simulink subsystem "patient_model"  (R2019b)
settings: Solver=VariableStepAuto  StartTime=0.0  StopTime=10.0  RelTol=1e-3
undefined symbols (not defined in the file): C_v_CO2_0, C_v_O2_0, Q_0
libraries: simulink x1
(part 1 of 2)
settings Model: Creator=RH  LastModifiedBy=RH

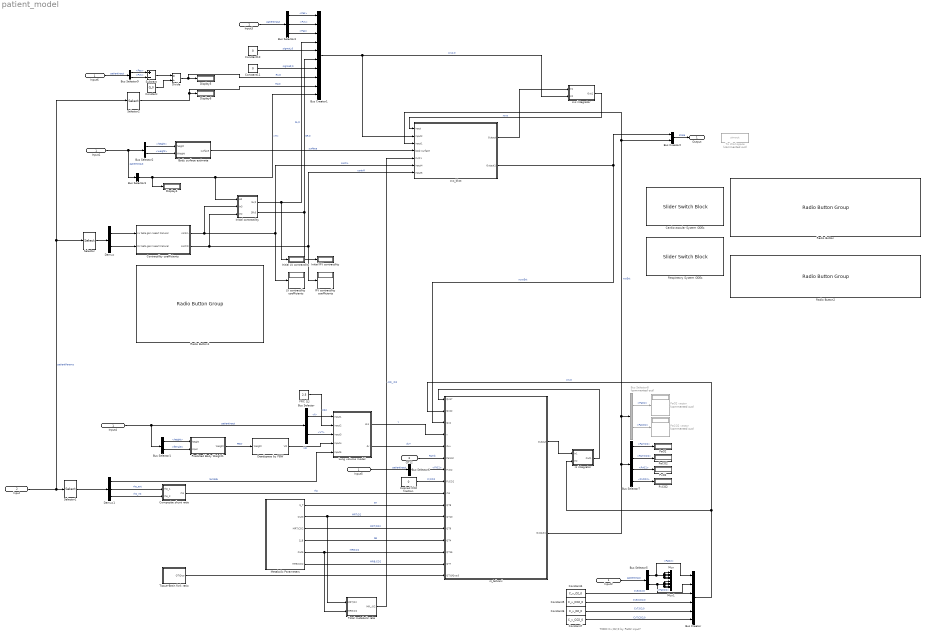
== system patient_model ==
  note: TODO Cv;O2;0 by PaO2 input?
  Input1 : Inport  OutDataTypeStr=Bus: PatientInput
  Input : Inport  Port=2  PortDimensions=6
  QT12 : Inport  Port=3  Unit=mmHg
  Body surface estimate : Subsystem  TreatAsAtomicUnit=on
  Bus Creator : BusCreator  Inputs=6  OutDataTypeStr=Bus: RespiratoryState
      settings: InheritFromInputs=off
  Bus Creator1 : BusCreator  Inputs=10  OutDataTypeStr=Bus: CardioVascularState
      settings: InheritFromInputs=off
  Bus Creator2 : BusCreator  Inputs=2  OutDataTypeStr=Bus: PatientState
      settings: InheritFromInputs=off
  Bus Selector : BusSelector  OutputSignals=f,VT
  Bus Selector1 : BusSelector  OutputSignals=height,female
  Bus Selector2 : BusSelector  OutputSignals=height,weight
  Bus Selector3 : BusSelector  OutputSignals=H
  Bus Selector4 : BusSelector  OutputSignals=Pas,Pvs,Pap
  Bus Selector5 : BusSelector  OutputSignals=PaO2,PaCO2
  Bus Selector6 : BusSelector  OutputSignals=FiO2
  Bus Selector7 : BusSelector  OutputSignals=PamO2,PamCO2,PvO2,PvCO2
  Bus Selector8 : BusSelector  Commented=on  OutputSignals=PaO2,PaCO2
  Bus Selector9 : BusSelector  OutputSignals=Pas,Pvs
  Cardiovascular System ODEs : SliderSwitchBlock
      settings: Values={{'Off', 'On'}, [0 1]}
  Composite shunt ratio : Subsystem
  Constant : Constant  Value=Q_0
  Constant10 : Constant  Value=0
  Constant11 : Constant  Value=0
  Constant4 : Constant  Value=C_v_O2_0
  Constant5 : Constant  Value=C_v_CO2_0
  Constant6 : Constant  Value=C_v_O2_0
  Constant7 : Constant  Value=C_v_CO2_0
  Contractility coefficients : Subsystem
  Deadspace by PBW : Subsystem  TreatAsAtomicUnit=on
  Demux : Demux  Outputs=2
  Demux1 : Demux  Outputs=3
  Display4 : Display
  Display5 : Display
  Display6 : Display
  Divide : Product  Inputs=*/
  FRC [L] : Constant  Value=2.5
  Initial LV contractility : Display
  Initial RV contractility : Display
  Initial contractility : Subsystem
  Input{2..6} (5 alike) : InportShadow  OutDataTypeStr=Bus: PatientInput
  Inspired CO2 fraction : Constant  Value=0
  LV contractility coefficients : Display
  Lung volume model : Subsystem  TreatAsAtomicUnit=on
  Metabolic Parameters : Subsystem
  Mux : Mux  Inputs=5
  Mux1 : Mux  Inputs=5
  PaCO2 : Display
  PaCO2 vector : Display  Commented=on
  PaO2 : Display
  PaO2 vector : Display  Commented=on
  Predicted Body Weight1 : Subsystem  TreatAsAtomicUnit=on
  PvCO2 : Display
  PvO2 : Display
  RV contractility coefficients : Display
  Radio Button : RadioButtonGroup  LabelPosition=Hide  SelectedLabel=ODE from [BKST (1.27)]: By Metabolic rates and Ca;O2  ButtonGroupName=Systemic vascular resistance: Calculation mode
      settings: Values={{'Constant', 'Linear relation from [BKST (1.24)]: By Cv;O2', 'ODE from [BKST (1.27)]: By Metabolic rates and Ca;O2'}, [0 1 2]}
  Radio Button1 : RadioButtonGroup  LabelPosition=Hide  SelectedLabel=from table 3.1 (healthy)  ButtonGroupName=Contractility coefficient selection (see [BKST] table 1.5)
      settings: Values={{'without QL measurements', 'with QL measurements', 'with QL measurements, "exact" gradients', 'from table 3.1 (healthy)', 'from table 3.1 (Heart Failure)'}, [1 2 3 4 5]}
  Radio Button2 : RadioButtonGroup  LabelPosition=Hide  SelectedLabel=Linear relationship with Heart Frequency (H)  ButtonGroupName=Heart Contractility: Calculation mode
      settings: Values={{'Linear relationship with Heart Frequency (H)', 'Second-order ODE'}, [0 1]}
  Respiratory System ODEs : SliderSwitchBlock
      settings: Values={{'Off', 'On'}, [0 1]}
  Selector : Selector  InputPortWidth=6  IndexOptions=Index vector (dialog)  Indices=[1 2]  OutputSizes=1
  Selector1 : Selector  InputPortWidth=6  IndexOptions=Index vector (dialog)  Indices=[3 4 5]  OutputSizes=1
  Selector2 : Selector  InputPortWidth=6  IndexOptions=Index vector (dialog)  Indices=[6]  OutputSizes=1
  Subtract : Sum  Inputs=+-
  Tissue-Brain fork ratio : Subsystem
  To Workspace : ToWorkspace  Commented=on  VariableName=simout  SaveFormat=Timeseries  SampleTime=-1
      settings: MaxDataPoints=1
  Total metabolic rate : Subsystem
  cvs integrator : Subsystem
  cvs_bkst : Subsystem
  rs integrator : Subsystem
  rs_tehrani : Subsystem  TreatAsAtomicUnit=on
  Output : Outport  OutDataTypeStr=Bus: PatientState
  wires:
  Lung volume model/2(dv) -> rs_tehrani/5(dv+)  "dv+"
  QT12/1 -> rs_tehrani/6(Pamb*)  "Pamb"
  Bus Selector/1 -> Lung volume model/1(Input1)  "<f>"
  FRC [L]/1 -> Lung volume model/2(Input2)  "FRC"
  Deadspace by PBW/1(VD) -> Lung volume model/4(Input4)  "VD"
  Bus Selector2/1 -> Body surface estimate/1(height)  "<height>"
  Predicted Body Weight1/1(Weight) -> Deadspace by PBW/1(Weight)  "PBW"
  Lung volume model/1(dv1) -> rs_tehrani/4(v)  "v"
  Bus Selector6/1 -> rs_tehrani/7(Fi;O2)  "<FiO2>"
  Inspired CO2 fraction/1 -> rs_tehrani/8(Fi;CO2)  "Fi;CO2"
  Composite shunt ratio/1(rho) -> rs_tehrani/9(rho)  "rho"
  Metabolic Parameters/1(S_T) -> rs_tehrani/10(QT8)  "ST"
  Metabolic Parameters/2(Out3) -> rs_tehrani/11(QT10), Total metabolic rate/1(MRT;O2)  "MRT;O2"
  Metabolic Parameters/3(MRT;CO2) -> rs_tehrani/12(QT9)  "MRT;CO2"
  Metabolic Parameters/4(S_B) -> rs_tehrani/13(QT4)  "SB"
  Metabolic Parameters/5(Out5) -> rs_tehrani/14(QT15), Total metabolic rate/2(MRB;O2)  "MRB;O2"
  Metabolic Parameters/6(MRB;CO2) -> rs_tehrani/15(QT7)  "MRB;CO2"
  Demux1/3 -> Composite shunt ratio/2(rho_2)  "rho_int"
  Demux1/2 -> Composite shunt ratio/1(rho_1)  "rho_ext"
  Tissue-Brain fork ratio/1(QT/Qco) -> rs_tehrani/16(QT;0/Qco;0)
  Bus Selector2/2 -> Body surface estimate/2(Weight)  "<weight>"
  Bus Selector3/1 -> Initial contractility/1(H0), Bus Creator1/10, Display4/1  "<H>"
  Body surface estimate/1(surface) -> cvs_bkst/4(body surface)  "surface"
  Demux1/1 -> Lung volume model/5(Input5)  "lambda"
  Constant4/1 -> Bus Creator/3  "CvB;O2;0"
  Constant5/1 -> Bus Creator/4  "CvB;CO2;0"
  Constant6/1 -> Bus Creator/5  "CvT;O2;0"
  Constant7/1 -> Bus Creator/6  "CvT;CO2;0"
  Bus Selector5/1 -> Mux/3, Mux/2, Mux/1, Mux/4, Mux/5, Bus Creator/1  "<PaO2>"
  rs_tehrani/1(Output) -> rs integrator/1(In1)
  Bus Creator/1 -> rs_tehrani/2(Qco2), rs integrator/2(In2)  "xrs;0"
  rs integrator/1(Out1) -> rs_tehrani/1(Qco7)
  Divide/1 -> Display5/1, Bus Creator1/8  "Rs;0"
  Initial contractility/2(SR;0) -> Bus Creator1/6, Initial RV contractility/1  "SR;0"
  Initial contractility/1(SL;0) -> Bus Creator1/4, Initial LV contractility/1  "SL;0"
  Constant11/1 -> Bus Creator1/7  "sigmaR;0"
  Demux/1 -> Contractility coefficients/1(LV beta gain (Heart Failure))
  Demux/2 -> Contractility coefficients/2(RV beta gain (Heart Failure))
  Bus Selector4/2 -> Bus Creator1/2  "<Pvs>"
  Selector2/1 -> Display6/1, Bus Creator1/9  "Rp;0"
  Total metabolic rate/1(MR_;O2) -> cvs_bkst/5(CvO1)  "-MR_;O2"
  Bus Creator1/1 -> cvs_bkst/2(Input2), cvs integrator/2(In2)  "xcvs;0"
  Constant10/1 -> Bus Creator1/5  "sigmaL;0"
  Bus Selector4/3 -> Bus Creator1/3  "<Pap>"
  Bus Selector4/1 -> Bus Creator1/1  "<Pas>"
  rs_tehrani/2(Output1) -> Bus Selector7/1, Bus Selector8/1, cvs_bkst/3(Input1), Bus Creator2/2  "xrsExt"
  cvs_bkst/1(Output) -> cvs integrator/1(In1)
  Contractility coefficients/2(contrR) -> Initial contractility/3(In2), RV contractility coefficients/1, cvs_bkst/7(Input5)  "contrR"
  Contractility coefficients/1(contrL) -> Initial contractility/2(In3), LV contractility coefficients/1, cvs_bkst/6(Input4)  "contrL"
  cvs integrator/1(Out1) -> cvs_bkst/1(Input)  "xcvs"
  cvs_bkst/2(Output1) -> rs_tehrani/3(Qco), Bus Creator2/1  "xcvsExt"
  Bus Creator2/1 -> Output/1  "state"
  Input1/1 -> Bus Selector3/1, Bus Selector2/1  "patientInput"
  Input4/1 -> Bus Selector/1, Bus Selector1/1  "patientInput"
  Input3/1 -> Bus Selector4/1  "patientInput"
  Bus Selector1/2 -> Predicted Body Weight1/2(Input)  "<female>"
  Bus Selector/2 -> Lung volume model/3(Input3)  "<VT>"
  Input2/1 -> Bus Selector5/1  "patientInput"
  Input5/1 -> Bus Selector6/1  "patientInput"
  Bus Selector7/1 -> PaO2/1  "<PamO2>"
  Bus Selector7/2 -> PaCO2/1  "<PamCO2>"
  Bus Selector7/3 -> PvO2/1  "<PvO2>"
  Bus Selector7/4 -> PvCO2/1  "<PvCO2>"
  Bus Selector5/2 -> Mux1/1, Mux1/2, Mux1/3, Mux1/4, Mux1/5, Bus Creator/2  "<PaCO2>"
  Bus Selector8/1 -> PaO2 vector/1  "<PaO2>"
  Bus Selector8/2 -> PaCO2 vector/1  "<PaCO2>"
  Bus Selector1/1 -> Predicted Body Weight1/1(height)  "<height>"
  Selector/1 -> Demux/1
  Selector1/1 -> Demux1/1
  Input/1 -> Selector1/1, Selector2/1, Selector/1  "patientParams"
  Input6/1 -> Bus Selector9/1  "patientInput"
  Bus Selector9/1 -> Subtract/1  "<Pas>"
  Bus Selector9/2 -> Subtract/2  "<Pvs>"
  Subtract/1 -> Divide/1
  Constant/1 -> Divide/2

== system patient_model/Body surface estimate ==
  note: s = 0.007184 w^0.425 h^0.725
      |
      | source: CVRS ch 1.6.1 [Du Bois’ formula (Keidl, 1985, p. 377)]
      | WolframAlpha
  height : Inport  Unit=m
  Weight : Inport  Port=2  Unit=kg
  Constant1 : Constant  Value=0.007184
  Constant2 : Constant  Value=0.725
  Constant3 : Constant  Value=0.425
  Gain : Gain  Gain=100
  Power : Math  Operator=pow  SignedPower=off  SaturateOnIntegerOverflow=on
  Power1 : Math  Operator=pow  SignedPower=off  SaturateOnIntegerOverflow=on
  Product2 : Product  Inputs=***
  surface : Outport  Unit=m^2
  wires:
  Gain/1 -> Power/1  "height [cm]"
  height/1 -> Gain/1  "height"
  Weight/1 -> Power1/1  "weight"
  Power/1 -> Product2/1
  Constant3/1 -> Power1/2
  Product2/1 -> surface/1  "surface"
  Constant1/1 -> Product2/3
  Constant2/1 -> Power/2
  Power1/1 -> Product2/2

== system patient_model/Composite shunt ratio ==
  rho_1 : Inport
  rho_2 : Inport  Port=2
  Add1 : Sum
  Constant : Constant
  Product : Product
  Subtract : Sum  Inputs=+-
  rho : Outport
  wires:
  Constant/1 -> Subtract/1
  rho_2/1 -> Product/1
  Subtract/1 -> Product/2
  Add1/1 -> rho/1  "rho"
  Product/1 -> Add1/2
  rho_1/1 -> Subtract/2, Add1/1

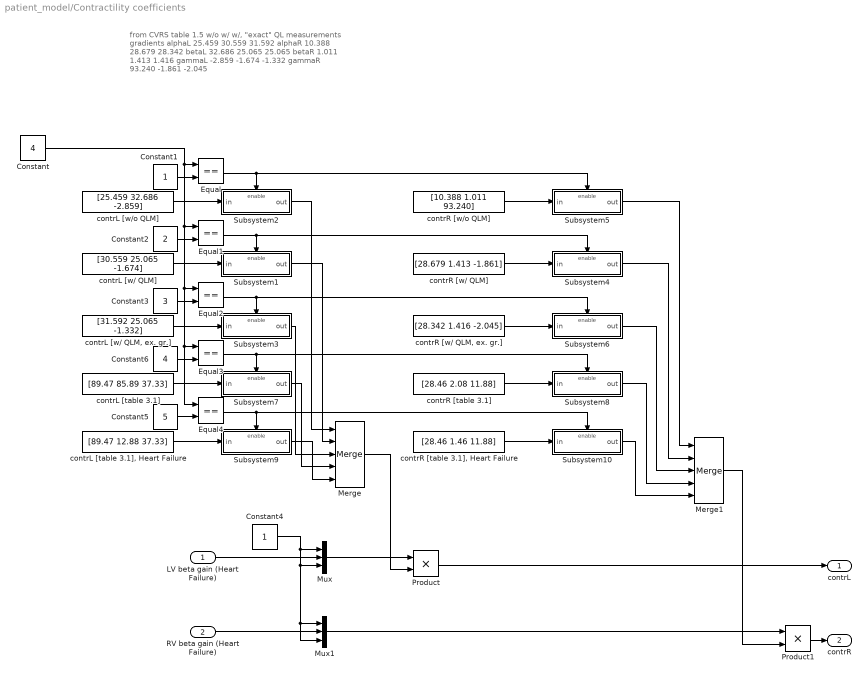
== system patient_model/Contractility coefficients ==
  note: from CVRS table 1.5
      | w/o w/ w/, "exact"
      | QL measurements gradients
      |
      | alphaL 25.459 30.559 31.592
      | alphaR 10.388 28.679 28.342
      | betaL 32.686 25.065 25.065
      | betaR 1.011 1.413 1.416
      | gammaL -2.859 -1.674 -1.332
      | gammaR 93.240 -1.861 -2.045
  LV beta gain (Heart Failure) : Inport
  RV beta gain (Heart Failure) : Inport  Port=2
  Constant : Constant  Value=4
  Constant1 : Constant
  Constant2 : Constant  Value=2
  Constant3 : Constant  Value=3
  Constant4 : Constant
  Constant5 : Constant  Value=5
  Constant6 : Constant  Value=4
  Equal{,1..4} (5 alike) : RelationalOperator  Operator===  OutDataTypeStr=boolean  RndMeth=Simplest
  Merge : Merge  Inputs=5
  Merge1 : Merge  Inputs=5
  Mux : Mux  Inputs=3
  Mux1 : Mux  Inputs=3
  Product : Product
  Product1 : Product
  Subsystem1 : Subsystem
  Subsystem10 : Subsystem
  Subsystem2 : Subsystem
  Subsystem3 : Subsystem
  Subsystem4 : Subsystem
  Subsystem5 : Subsystem
  Subsystem6 : Subsystem
  Subsystem7 : Subsystem
  Subsystem8 : Subsystem
  Subsystem9 : Subsystem
  contrL [table 3.1] : Constant  Value=[89.47 85.89 37.33]
  "contrL [table 3.1], Heart Failure" : Constant  Value=[89.47 12.88 37.33]
  "contrL [w/ QLM, ex. gr.]" : Constant  Value=[31.592 25.065 -1.332]
  contrL [w/ QLM] : Constant  Value=[30.559 25.065 -1.674]
  contrL [w/o QLM] : Constant  Value=[25.459 32.686 -2.859]
  contrR [table 3.1] : Constant  Value=[28.46 2.08 11.88]
  "contrR [table 3.1], Heart Failure" : Constant  Value=[28.46 1.46 11.88]
  "contrR [w/ QLM, ex. gr.]" : Constant  Value=[28.342 1.416 -2.045]
  contrR [w/ QLM] : Constant  Value=[28.679 1.413 -1.861]
  contrR [w/o QLM] : Constant  Value=[10.388 1.011 93.240]
  contrL : Outport  OutDataTypeStr=double  PortDimensions=3
  contrR : Outport  Port=2  OutDataTypeStr=double  PortDimensions=3
  wires:
  "contrL [table 3.1], Heart Failure"/1 -> Subsystem9/1(in)
  Constant5/1 -> Equal4/2
  Equal4/1 -> Subsystem10/Enable, Subsystem9/Enable
  Subsystem9/1(out) -> Merge/5
  Subsystem10/1(out) -> Merge1/5
  "contrR [table 3.1], Heart Failure"/1 -> Subsystem10/1(in)
  contrR [table 3.1]/1 -> Subsystem8/1(in)
  Subsystem8/1(out) -> Merge1/4
  Subsystem7/1(out) -> Merge/4
  Equal3/1 -> Subsystem7/Enable, Subsystem8/Enable
  Constant6/1 -> Equal3/2
  contrL [table 3.1]/1 -> Subsystem7/1(in)
  Product1/1 -> contrR/1
  Product/1 -> contrL/1
  Merge1/1 -> Product1/2
  Mux1/1 -> Product1/1
  Merge/1 -> Product/2
  Mux/1 -> Product/1
  Constant4/1 -> Mux/1, Mux/3, Mux1/3, Mux1/1
  Subsystem6/1(out) -> Merge1/3
  Subsystem4/1(out) -> Merge1/2
  Subsystem5/1(out) -> Merge1/1
  "contrR [w/ QLM, ex. gr.]"/1 -> Subsystem6/1(in)
  contrR [w/ QLM]/1 -> Subsystem4/1(in)
  contrR [w/o QLM]/1 -> Subsystem5/1(in)
  Subsystem3/1(out) -> Merge/3
  Subsystem2/1(out) -> Merge/1
  Subsystem1/1(out) -> Merge/2
  Constant3/1 -> Equal2/2
  Equal2/1 -> Subsystem3/Enable, Subsystem6/Enable
  Constant2/1 -> Equal1/2
  Equal1/1 -> Subsystem1/Enable, Subsystem4/Enable
  Equal/1 -> Subsystem2/Enable, Subsystem5/Enable
  "contrL [w/ QLM, ex. gr.]"/1 -> Subsystem3/1(in)
  contrL [w/ QLM]/1 -> Subsystem1/1(in)
  contrL [w/o QLM]/1 -> Subsystem2/1(in)
  Constant1/1 -> Equal/2
  Constant/1 -> Equal/1, Equal1/1, Equal2/1, Equal3/1, Equal4/1
  RV beta gain (Heart Failure)/1 -> Mux1/2
  LV beta gain (Heart Failure)/1 -> Mux/2

== system patient_model/Deadspace by PBW ==
  Weight : Inport  Unit=kg
  Constant1 : Constant  Value=0.0026
  Product2 : Product
  VD : Outport  Unit=L
  wires:
  Weight/1 -> Product2/1  "PBW"
  Product2/1 -> VD/1  "VD"
  Constant1/1 -> Product2/2

== system patient_model/Initial contractility ==
  H0 : Inport  Unit=1/min
  In3 : Inport  Port=2  OutDataTypeStr=double  PortDimensions=3
  In2 : Inport  Port=3  OutDataTypeStr=double  PortDimensions=3
  Demux : Demux  Outputs=2
  Demux1 : Demux  Outputs=2
  Product : Product  Inputs=*/*
  Product1 : Product  Inputs=*/*
  Selector : Selector  InputPortWidth=3  IndexOptions=Index vector (dialog)  Indices=[1 2]  OutputSizes=1
  Selector1 : Selector  InputPortWidth=3  IndexOptions=Index vector (dialog)  Indices=[1 2]  OutputSizes=1
  SL;0 : Outport  Unit=mmHg
  SR;0 : Outport  Port=2  Unit=mmHg
  wires:
  Selector1/1 -> Demux1/1
  In2/1 -> Selector1/1  "contrR"
  Demux/2 -> Product1/3  "betaL"
  In3/1 -> Selector/1  "contrL"
  H0/1 -> Product/1, Product1/1  "H0"
  Demux/1 -> Product1/2  "alphaL"
  Selector/1 -> Demux/1
  Demux1/1 -> Product/2  "alphaR"
  Product/1 -> SR;0/1  "SR;0"
  Demux1/2 -> Product/3  "betaR"
  Product1/1 -> SL;0/1  "SL;0"

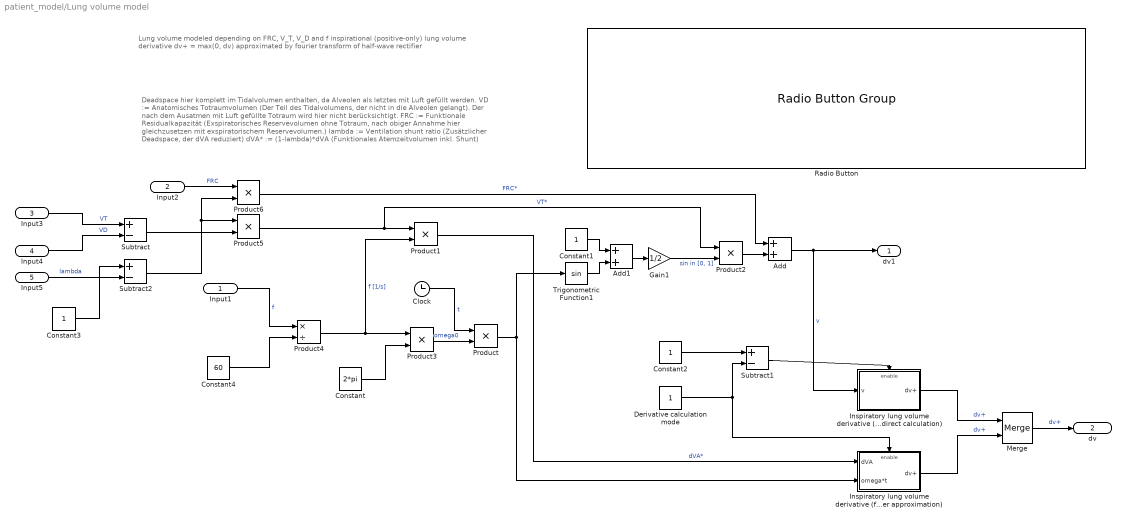
== system patient_model/Lung volume model ==
  note: Lung volume modeled depending on FRC, V_T, V_D and f
      |
      | inspirational (positive-only) lung volume derivative dv+ = max(0, dv) approximated by fourier transform of half-wave rectifier
  note: Deadspace hier komplett im Tidalvolumen enthalten, da Alveolen als letztes mit Luft gefüllt werden.
      |
      | VD := Anatomisches Totraumvolumen (Der Teil des Tidalvolumens, der nicht in die Alveolen gelangt).
      | 	Der nach dem Ausatmen mit Luft gefüllte Totraum wird hier nicht berücksichtigt.
      | FRC := Funktionale Residualkapazität (Exspiratorisches Reservevolumen ohne Totraum,
      | 	nach obiger Annahme hier gleichzusetzen mit exspiratorischem Reservevolumen.)
      | lambda := Ventilation shunt ratio (Zusätzlicher Deadspace, der dVA reduziert)
      | dVA* := (1-lambda)*dVA (Funktionales Atemzeitvolumen inkl. Shunt)
  Input1 : Inport  Unit=1/min
  Input2 : Inport  Port=2  Unit=L
  Input3 : Inport  Port=3  Unit=L
  Input4 : Inport  Port=4  Unit=L
  Input5 : Inport  Port=5  OutMin=0  OutMax=1  Unit=1
  Add : Sum
  Add1 : Sum
  Clock : Clock
  Constant : Constant  Value=2*pi
  Constant1 : Constant
  Constant2 : Constant
  Constant3 : Constant
  Constant4 : Constant  Value=60
  Derivative calculation mode : Constant
  Gain1 : Gain  Gain=1/2
  Inspiratory lung volume derivative (direct calculation) : Subsystem
  Inspiratory lung volume derivative (fourier approximation) : Subsystem
  Merge : Merge
  Product{,1..3,5..6} (6 alike) : Product
  Product4 : Product  Inputs=*/
  Radio Button : RadioButtonGroup  SelectedLabel=Fourier approximation (continuous)  ButtonGroupName=Select mode
      settings: Values={{'Direct calculation (with discontinuities)', 'Fourier approximation (continuous)'}, [0 1]}
  Subtract : Sum  Inputs=+-
  Subtract1 : Sum  Inputs=+-
  Subtract2 : Sum  Inputs=+-
  Trigonometric Function1 : Trigonometry
  dv1 : Outport  Unit=L
  dv : Outport  Port=2  Unit=L/s
  wires:
  Input2/1 -> Product6/1  "FRC"
  Subtract2/1 -> Product5/1, Product6/2
  Subtract/1 -> Product5/2
  Constant3/1 -> Subtract2/1
  Input5/1 -> Subtract2/2  "lambda"
  Subtract1/1 -> Inspiratory lung volume derivative (direct calculation)/Enable
  Merge/1 -> dv/1  "dv+"
  Inspiratory lung volume derivative (direct calculation)/1(dv+) -> Merge/1  "dv+"
  Derivative calculation mode/1 -> Inspiratory lung volume derivative (fourier approximation)/Enable, Subtract1/2
  Constant2/1 -> Subtract1/1
  Inspiratory lung volume derivative (fourier approximation)/1(dv+) -> Merge/2  "dv+"
  Product1/1 -> Inspiratory lung volume derivative (fourier approximation)/1(dVA)  "dVA*"
  Product5/1 -> Product2/1, Product1/1  "VT*"
  Gain1/1 -> Product2/2  "sin in [0, 1]"
  Input1/1 -> Product4/1  "f"
  Constant4/1 -> Product4/2
  Product/1 -> Trigonometric Function1/1, Inspiratory lung volume derivative (fourier approximation)/2(omega*t)
  Constant/1 -> Product3/2
  Input4/1 -> Subtract/2  "VD"
  Input3/1 -> Subtract/1  "VT"
  Constant1/1 -> Add1/1
  Add1/1 -> Gain1/1
  Add/1 -> dv1/1, Inspiratory lung volume derivative (direct calculation)/1(v)  "v"
  Product6/1 -> Add/1  "FRC*"
  Product2/1 -> Add/2
  Trigonometric Function1/1 -> Add1/2
  Clock/1 -> Product/1  "t"
  Product4/1 -> Product1/2, Product3/1  "f [1/s]"
  Product3/1 -> Product/2  "omega0"

== system patient_model/Metabolic Parameters ==
  note: S_T = 50 lit (Fincham-Tehrani)
      | S_T = 13 lit (Tehrani DSS)
  Equivalent gas storage (body tissue) [lit] : Constant  Value=13
  Equivalent gas storage (brain) [lit] : Constant  Value=1.1
  "Metabolic rate (CO2, body tissue) [lit/s]" : Constant  Value=0.00287
  "Metabolic rate (CO2, brain) [lit/s]" : Constant  Value=0.0009
  "Metabolic rate (O2, body tissue, positive) [lit/s]" : Constant  Value=0.00352
  "Metabolic rate (O2, brain, positive) [lit/s]" : Constant  Value=0.000925
  Multiply : Gain  Gain=-1
  Multiply1 : Gain  Gain=-1
  S_T : Outport  Unit=L
  Out3 : Outport  Port=2  Unit=L/s
  MRT;CO2 : Outport  Port=3  Unit=L/s
  S_B : Outport  Port=4  Unit=L
  Out5 : Outport  Port=5  Unit=L/s
  MRB;CO2 : Outport  Port=6  Unit=L/s
  wires:
  "Metabolic rate (CO2, brain) [lit/s]"/1 -> MRB;CO2/1  "MRB;CO2"
  Equivalent gas storage (brain) [lit]/1 -> S_B/1  "S_B"
  Multiply/1 -> Out5/1  "MRB;O2"
  Multiply1/1 -> Out3/1  "MRT;O2"
  "Metabolic rate (CO2, body tissue) [lit/s]"/1 -> MRT;CO2/1  "MRT;CO2"
  "Metabolic rate (O2, brain, positive) [lit/s]"/1 -> Multiply/1  "-MRB;O2"
  "Metabolic rate (O2, body tissue, positive) [lit/s]"/1 -> Multiply1/1  "-MRT;O2"
  Equivalent gas storage (body tissue) [lit]/1 -> S_T/1  "S_T"

== system patient_model/Predicted Body Weight1 ==
  note: Predicted body weight
      | Source: Ventilation with lower tidal volumes [...], page 3
  height : Inport  Unit=m
  Input : Inport  Port=2  OutDataTypeStr=boolean
  Add4 : Sum  Inputs=+-
  Constant1 : Constant  Value=1.524
  Constant3 : Constant  Value=0
  Gain : Gain  Gain=91
  IfThenElse : Subsystem
  Max : MinMax  Function=max  Inputs=2
  Subtract1 : Sum
  female : Constant  Value=45.5
  male : Constant  Value=50
  Weight : Outport  Unit=kg
  wires:
  IfThenElse/1(out) -> Subtract1/2
  male/1 -> IfThenElse/3(else)
  female/1 -> IfThenElse/2(then)
  Input/1 -> IfThenElse/1(if)  "female"
  Add4/1 -> Max/1
  Subtract1/1 -> Weight/1  "PBW"
  height/1 -> Add4/1  "height"
  Constant3/1 -> Max/2
  Gain/1 -> Subtract1/1
  Constant1/1 -> Add4/2
  Max/1 -> Gain/1

== system patient_model/Tissue-Brain fork ratio ==
  note: Tissue-Brain fork ratio
      | Use blood flow rates from [TehraniAbbasi] to calculate fork ratio
  Add : Sum
  Blood flow in body tissue [lit/s] : Constant  Value=0.07083
  Blood flow in brain [lit/s] : Constant  Value=0.0125
  Divide : Product  Inputs=*/
  QT/Qco : Outport  Unit=1
  wires:
  Blood flow in body tissue [lit/s]/1 -> Add/1, Divide/1  "QT;0"
  Blood flow in brain [lit/s]/1 -> Add/2  "QB;0"
  Add/1 -> Divide/2  "Qco;0"
  Divide/1 -> QT/Qco/1  "QT/Qco"

== system patient_model/Total metabolic rate ==
  MRT;O2 : Inport  Unit=L/s
  MRB;O2 : Inport  Port=2  Unit=L/s
  Add : Sum  Inputs=--
  Constant : Constant  Value=60
  Product : Product
  MR_;O2 : Outport  Unit=L/min
  wires:
  MRT;O2/1 -> Add/1
  Add/1 -> Product/1
  MRB;O2/1 -> Add/2
  Constant/1 -> Product/2
  Product/1 -> MR_;O2/1  "-MR_;O2"

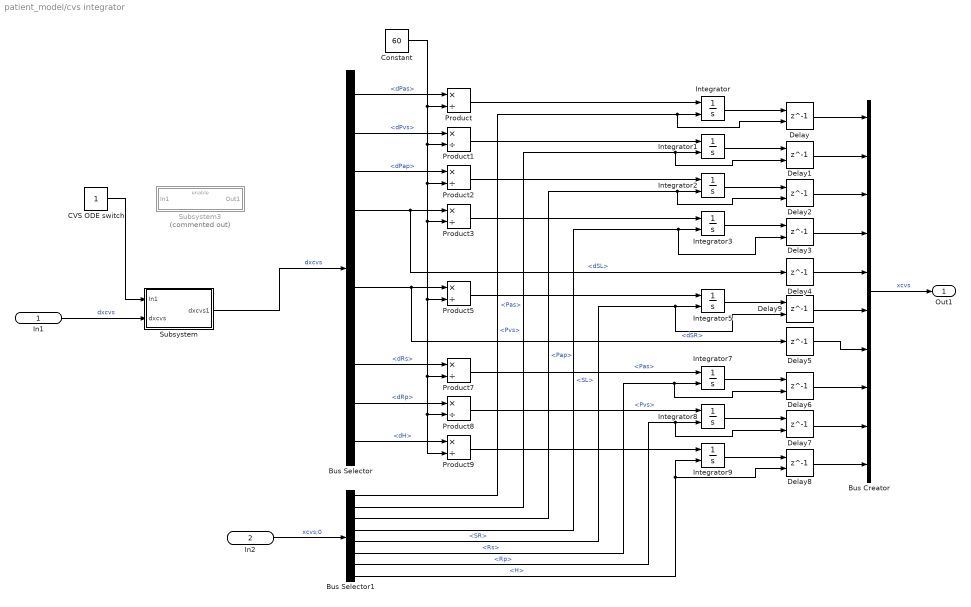
== system patient_model/cvs integrator ==
  In1 : Inport  OutDataTypeStr=Bus: CardioVascularStateDerivative
  In2 : Inport  Port=2  OutDataTypeStr=Bus: CardioVascularState
  Bus Creator : BusCreator  Inputs=10  OutDataTypeStr=Bus: CardioVascularState
      settings: InheritFromInputs=off
  Bus Selector : BusSelector  OutputSignals=dPas,dPvs,dPap,dSL,dsigmaL,dSR,dsigmaR,dRs,dRp,dH
  Bus Selector1 : BusSelector  OutputSignals=Pas,Pvs,Pap,SL,SR,Rs,Rp,H
  CVS ODE switch : Constant
  Constant : Constant  Value=60
  Delay{,1..3,6..9} (8 alike) : Delay  DelayLength=1  InitialConditionSource=Input port
      settings: InputPortMap=u0,p4
  Delay4 : Delay  DelayLength=1
  Delay5 : Delay  DelayLength=1
  Integrator{,1..3,5,7..9} (8 alike) : Integrator  InitialConditionSource=external
  Product{,1..3,5,7..9} (8 alike) : Product  Inputs=*/
  Subsystem : Subsystem
  Subsystem3 : Subsystem  Commented=on
  Out1 : Outport  OutDataTypeStr=Bus: CardioVascularState
  wires:
  CVS ODE switch/1 -> Subsystem/1(In1)
  In1/1 -> Subsystem/2(dxcvs)  "dxcvs"
  Subsystem/1(dxcvs1) -> Bus Selector/1  "dxcvs"
  Delay9/1 -> Bus Creator/6
  Integrator5/1 -> Delay9/1
  Delay8/1 -> Bus Creator/10
  Delay7/1 -> Bus Creator/9
  Delay6/1 -> Bus Creator/8
  Delay/1 -> Bus Creator/1
  Delay1/1 -> Bus Creator/2
  Delay2/1 -> Bus Creator/3
  Delay3/1 -> Bus Creator/4
  Delay4/1 -> Bus Creator/5
  Bus Selector1/8 -> Integrator9/2, Delay8/2  "<H>"
  Product7/1 -> Integrator7/1  "<Pas>"
  Product8/1 -> Integrator8/1  "<Pvs>"
  Integrator7/1 -> Delay6/1
  Integrator8/1 -> Delay7/1
  Integrator9/1 -> Delay8/1
  Delay5/1 -> Bus Creator/7
  Integrator3/1 -> Delay3/1
  Integrator2/1 -> Delay2/1
  Integrator1/1 -> Delay1/1
  Integrator/1 -> Delay/1
  Bus Selector1/7 -> Integrator8/2, Delay7/2  "<Rp>"
  Bus Selector1/6 -> Integrator7/2, Delay6/2  "<Rs>"
  Bus Selector1/5 -> Integrator5/2, Delay9/2  "<SR>"
  Bus Selector1/4 -> Integrator3/2, Delay3/2  "<SL>"
  Bus Selector1/3 -> Integrator2/2, Delay2/2  "<Pap>"
  Bus Selector1/2 -> Integrator1/2, Delay1/2  "<Pvs>"
  Bus Selector1/1 -> Integrator/2, Delay/2  "<Pas>"
  Bus Selector/10 -> Product9/1  "<dH>"
  Bus Selector/9 -> Product8/1  "<dRp>"
  Bus Selector/8 -> Product7/1  "<dRs>"
  Bus Selector/6 -> Product5/1, Delay5/1  "<dSR>"
  Product5/1 -> Integrator5/1
  Product9/1 -> Integrator9/1
  Bus Selector/4 -> Product3/1, Delay4/1  "<dSL>"
  Product3/1 -> Integrator3/1
  Bus Selector/2 -> Product1/1  "<dPvs>"
  Bus Selector/3 -> Product2/1  "<dPap>"
  Product2/1 -> Integrator2/1
  Product1/1 -> Integrator1/1
  Product/1 -> Integrator/1
  Constant/1 -> Product/2, Product1/2, Product2/2, Product3/2, Product5/2, Product7/2, Product8/2, Product9/2
  Bus Selector/1 -> Product/1  "<dPas>"
  Bus Creator/1 -> Out1/1  "xcvs"
  In2/1 -> Bus Selector1/1  "xcvs;0"

== system patient_model/cvs_bkst ==
  Input : Inport  OutDataTypeStr=Bus: CardioVascularState
  Input2 : Inport  Port=2  OutDataTypeStr=Bus: CardioVascularState
  Input1 : Inport  Port=3  OutDataTypeStr=Bus: RespiratoryStateExtended
  body surface : Inport  Port=4  Unit=m^2
  CvO1 : Inport  Port=5  Unit=L/min
  Input4 : Inport  Port=6  OutDataTypeStr=double  PortDimensions=3
  Input5 : Inport  Port=7  OutDataTypeStr=double  PortDimensions=3
  Input3 : InportShadow  OutDataTypeStr=Bus: CardioVascularState
  ODEs : Subsystem
  calculations : Subsystem  ReferencedSubsystem=cvs_calculations
  initial calculations : Subsystem  Commented=on  ReferencedSubsystem=cvs_calculations
  Output : Outport  OutDataTypeStr=Bus: CardioVascularStateDerivative
  Output1 : Outport  Port=2  OutDataTypeStr=Bus: CardioVascularStateExtended
  wires:
  calculations/2 -> ODEs/2(c_)
  ODEs/1(dxcvs [/min]) -> Output/1  "dxcvs"
  calculations/1 -> ODEs/1(xcvsExt), Output1/1  "xcvsExt"
  Input2/1 -> initial calculations/1  "xcvs;0"
  CvO1/1 -> ODEs/7(CvO1)  "-MR_;O2"
  Input1/1 -> ODEs/6(Input1)  "xrsExt"
  Input3/1 -> ODEs/5(Input)  "xcvs"
  Input5/1 -> ODEs/4(Input5)  "contrR"
  Input4/1 -> ODEs/3(Input4)  "contrL"
  body surface/1 -> calculations/2, initial calculations/2  "surface"
  Input/1 -> calculations/1  "xcvs"

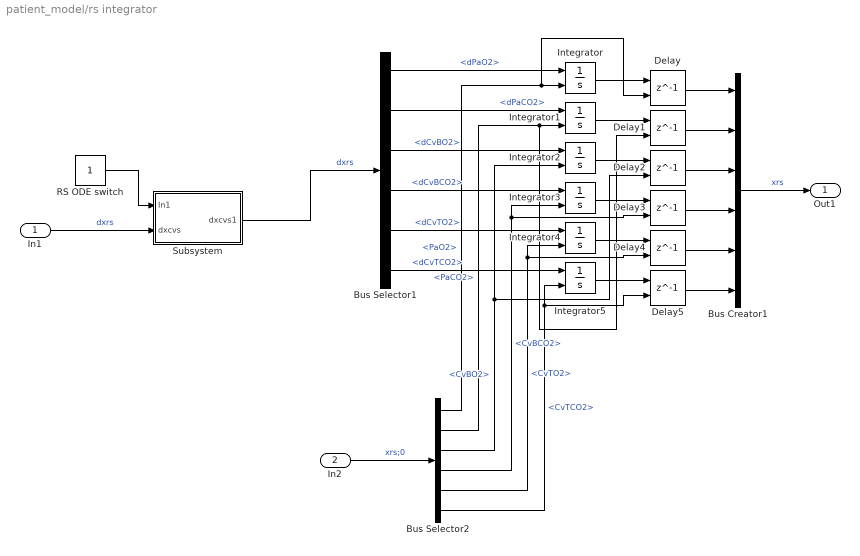
== system patient_model/rs integrator ==
  In1 : Inport  OutDataTypeStr=Bus: RespiratoryStateDerivative
  In2 : Inport  Port=2  OutDataTypeStr=Bus: RespiratoryState
  Bus Creator1 : BusCreator  Inputs=6  OutDataTypeStr=Bus: RespiratoryState
      settings: InheritFromInputs=off
  Bus Selector1 : BusSelector  OutputSignals=dPaO2,dPaCO2,dCvBO2,dCvBCO2,dCvTO2,dCvTCO2
  Bus Selector2 : BusSelector  OutputSignals=PaO2,PaCO2,CvBO2,CvBCO2,CvTO2,CvTCO2
  Delay{,1..5} (6 alike) : Delay  DelayLength=1  InitialConditionSource=Input port
      settings: InputPortMap=u0,p4
  Integrator{,1..5} (6 alike) : Integrator  InitialConditionSource=external
  RS ODE switch : Constant
  Subsystem : Subsystem
  Out1 : Outport  OutDataTypeStr=Bus: RespiratoryState
  wires:
  In1/1 -> Subsystem/2(dxcvs)  "dxrs"
  RS ODE switch/1 -> Subsystem/1(In1)
  Subsystem/1(dxcvs1) -> Bus Selector1/1  "dxrs"
  In2/1 -> Bus Selector2/1  "xrs;0"
  Bus Creator1/1 -> Out1/1  "xrs"
  Bus Selector1/2 -> Integrator1/1  "<dPaCO2>"
  Bus Selector1/6 -> Integrator5/1  "<dCvTCO2>"
  Bus Selector1/1 -> Integrator/1  "<dPaO2>"
  Delay/1 -> Bus Creator1/1
  Delay3/1 -> Bus Creator1/4
  Integrator3/1 -> Delay3/1
  Delay5/1 -> Bus Creator1/6
  Bus Selector2/5 -> Integrator4/2, Delay4/2  "<CvTO2>"
  Delay2/1 -> Bus Creator1/3
  Delay4/1 -> Bus Creator1/5
  Bus Selector1/5 -> Integrator4/1  "<dCvTO2>"
  Delay1/1 -> Bus Creator1/2
  Bus Selector2/4 -> Integrator3/2, Delay3/2  "<CvBCO2>"
  Bus Selector1/3 -> Integrator2/1  "<dCvBO2>"
  Integrator5/1 -> Delay5/1
  Integrator1/1 -> Delay1/1
  Bus Selector1/4 -> Integrator3/1  "<dCvBCO2>"
  Integrator2/1 -> Delay2/1
  Integrator4/1 -> Delay4/1
  Bus Selector2/2 -> Integrator1/2, Delay1/2  "<PaCO2>"
  Bus Selector2/1 -> Integrator/2, Delay/2  "<PaO2>"
  Bus Selector2/6 -> Integrator5/2, Delay5/2  "<CvTCO2>"
  Bus Selector2/3 -> Delay2/2, Integrator2/2  "<CvBO2>"
  Integrator/1 -> Delay/1

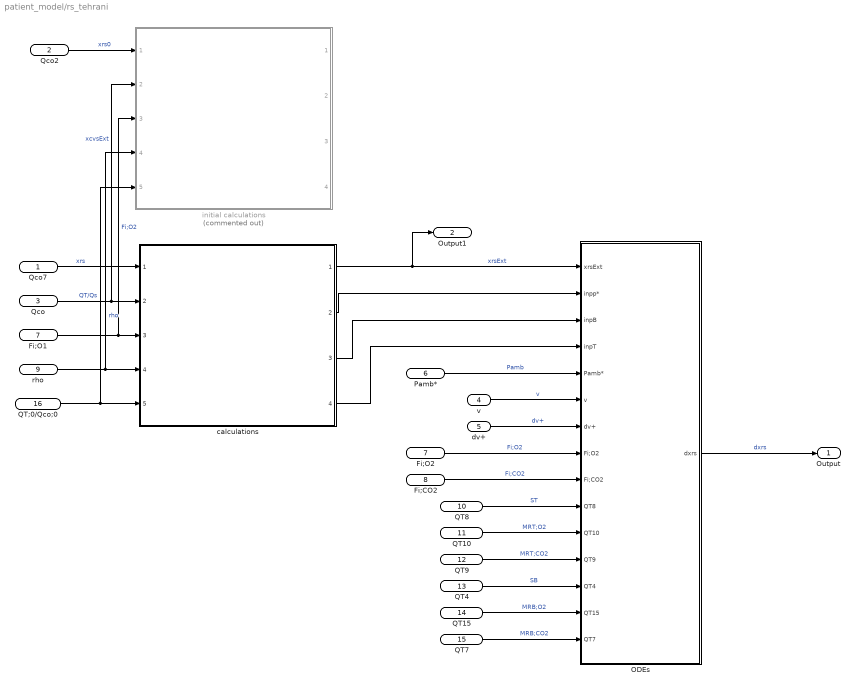
== system patient_model/rs_tehrani ==
  Qco7 : Inport  OutDataTypeStr=Bus: RespiratoryState  Unit=liter/minute
  Qco2 : Inport  Port=2  OutDataTypeStr=Bus: RespiratoryState  Unit=liter/minute
  Qco : Inport  Port=3  OutDataTypeStr=Bus: CardioVascularStateExtended  Unit=liter/minute
  v : Inport  Port=4  Unit=L
  dv+ : Inport  Port=5  Unit=liter/second
  Pamb* : Inport  Port=6  Unit=mmHg
  Fi;O2 : Inport  Port=7  Unit=1
  Fi;CO2 : Inport  Port=8  Unit=1
  rho : Inport  Port=9  Unit=1
  QT8 : Inport  Port=10  Unit=liter
  QT10 : Inport  Port=11  Unit=liter/second
  QT9 : Inport  Port=12  Unit=liter/s
  QT4 : Inport  Port=13  Unit=L
  QT15 : Inport  Port=14  Unit=liter/second
  QT7 : Inport  Port=15  Unit=liter/s
  QT;0/Qco;0 : Inport  Port=16  Unit=1
  Fi;O1 : InportShadow  Port=7  Unit=1
  ODEs : Subsystem
  calculations : Subsystem  ReferencedSubsystem=tehrani_rs_calculations
  initial calculations : Subsystem  Commented=on  ReferencedSubsystem=tehrani_rs_calculations
  Output : Outport  OutDataTypeStr=Bus: RespiratoryStateDerivative
  Output1 : Outport  Port=2  OutDataTypeStr=Bus: RespiratoryStateExtended
  wires:
  ODEs/1(dxrs) -> Output/1  "dxrs"
  QT7/1 -> ODEs/15(QT7)  "MRB;CO2"
  QT15/1 -> ODEs/14(QT15)  "MRB;O2"
  QT4/1 -> ODEs/13(QT4)  "SB"
  QT9/1 -> ODEs/12(QT9)  "MRT;CO2"
  QT10/1 -> ODEs/11(QT10)  "MRT;O2"
  calculations/4 -> ODEs/4(inpT)
  QT8/1 -> ODEs/10(QT8)  "ST"
  calculations/3 -> ODEs/3(inpB)
  calculations/2 -> ODEs/2(inpp*)
  Fi;CO2/1 -> ODEs/9(Fi;CO2)  "Fi;CO2"
  Fi;O2/1 -> ODEs/8(Fi;O2)  "Fi;O2"
  dv+/1 -> ODEs/7(dv+)  "dv+"
  v/1 -> ODEs/6(v)  "v"
  Pamb*/1 -> ODEs/5(Pamb*)  "Pamb"
  Qco2/1 -> initial calculations/1  "xrs0"
  Qco7/1 -> calculations/1  "xrs"
  QT;0/Qco;0/1 -> calculations/5, initial calculations/5  "QT/Qs"
  rho/1 -> calculations/4, initial calculations/4  "rho"
  Fi;O1/1 -> calculations/3, initial calculations/3  "Fi;O2"
  Qco/1 -> calculations/2, initial calculations/2  "xcvsExt"
  calculations/1 -> ODEs/1(xrsExt), Output1/1  "xrsExt"

== system patient_model/Contractility coefficients/Subsystem1 ==
  in : Inport  OutDataTypeStr=double  PortDimensions=3
  Enable : EnablePort
  out : Outport  OutDataTypeStr=double  PortDimensions=3
  wires:
  in/1 -> out/1

== system patient_model/Contractility coefficients/Subsystem10 ==
  in : Inport  OutDataTypeStr=double  PortDimensions=3
  Enable : EnablePort
  out : Outport  OutDataTypeStr=double  PortDimensions=3
  wires:
  in/1 -> out/1

== system patient_model/Contractility coefficients/Subsystem2 ==
  in : Inport  OutDataTypeStr=double  PortDimensions=3
  Enable : EnablePort
  out : Outport  OutDataTypeStr=double  PortDimensions=3
  wires:
  in/1 -> out/1

== system patient_model/Contractility coefficients/Subsystem3 ==
  in : Inport  OutDataTypeStr=double  PortDimensions=3
  Enable : EnablePort
  out : Outport  OutDataTypeStr=double  PortDimensions=3
  wires:
  in/1 -> out/1

== system patient_model/Contractility coefficients/Subsystem4 ==
  in : Inport  OutDataTypeStr=double  PortDimensions=3
  Enable : EnablePort
  out : Outport  OutDataTypeStr=double  PortDimensions=3
  wires:
  in/1 -> out/1

== system patient_model/Contractility coefficients/Subsystem5 ==
  in : Inport  OutDataTypeStr=double  PortDimensions=3
  Enable : EnablePort
  out : Outport  OutDataTypeStr=double  PortDimensions=3
  wires:
  in/1 -> out/1

== system patient_model/Contractility coefficients/Subsystem6 ==
  in : Inport  OutDataTypeStr=double  PortDimensions=3
  Enable : EnablePort
  out : Outport  OutDataTypeStr=double  PortDimensions=3
  wires:
  in/1 -> out/1

== system patient_model/Contractility coefficients/Subsystem7 ==
  in : Inport  OutDataTypeStr=double  PortDimensions=3
  Enable : EnablePort
  out : Outport  OutDataTypeStr=double  PortDimensions=3
  wires:
  in/1 -> out/1

== system patient_model/Contractility coefficients/Subsystem8 ==
  in : Inport  OutDataTypeStr=double  PortDimensions=3
  Enable : EnablePort
  out : Outport  OutDataTypeStr=double  PortDimensions=3
  wires:
  in/1 -> out/1

== system patient_model/Contractility coefficients/Subsystem9 ==
  in : Inport  OutDataTypeStr=double  PortDimensions=3
  Enable : EnablePort
  out : Outport  OutDataTypeStr=double  PortDimensions=3
  wires:
  in/1 -> out/1

== system patient_model/Lung volume model/Inspiratory lung volume derivative (direct calculation) ==
  v : Inport
  Enable : EnablePort
  Constant3 : Constant  Value=0
  Derivative : Derivative
  Max : MinMax  Function=max  Inputs=2
  dv+ : Outport
  wires:
  Derivative/1 -> Max/1
  Max/1 -> dv+/1  "dv+"
  v/1 -> Derivative/1
  Constant3/1 -> Max/2

== system patient_model/Lung volume model/Inspiratory lung volume derivative (fourier approximation) ==
  dVA : Inport
  omega*t : Inport  Port=2
  Enable : EnablePort
  Add2 : Sum
  Gain : Gain  Gain=pi
  Half-wave rectifier : Subsystem
  zero-prevention threshold : Constant  Value=0.01
  dv+ : Outport
  wires:
  dVA/1 -> Half-wave rectifier/1((d)VA)
  Gain/1 -> Add2/1
  Add2/1 -> dv+/1  "dv+"
  Half-wave rectifier/1(out) -> Gain/1
  zero-prevention threshold/1 -> Add2/2
  omega*t/1 -> Half-wave rectifier/2(2pift)

== system patient_model/Predicted Body Weight1/IfThenElse ==
  if : Inport  OutDataTypeStr=boolean
  then : Inport  Port=2
  else : Inport  Port=3
  Merge : Merge
  NOT : Logic  Operator=NOT  IconShape=distinctive  AllPortsSameDT=off  OutDataTypeStr=boolean
  Subsystem1 : Subsystem
  Subsystem2 : Subsystem
  out : Outport
  wires:
  Merge/1 -> out/1
  NOT/1 -> Subsystem2/Enable
  Subsystem1/1(out) -> Merge/1
  else/1 -> Subsystem2/1(in)
  if/1 -> Subsystem1/Enable, NOT/1
  Subsystem2/1(out) -> Merge/2
  then/1 -> Subsystem1/1(in)

== system patient_model/cvs integrator/Subsystem ==
  In1 : Inport
  dxcvs : Inport  Port=2
  Bus Creator1 : BusCreator  Inputs=10  OutDataTypeStr=Bus: CardioVascularStateDerivative
      settings: InheritFromInputs=off
  Bus to Vector : BusToVector
  Demux1 : Demux  Outputs=10
  Product : Product
  dxcvs1 : Outport
  wires:
  dxcvs/1 -> Bus to Vector/1  "dxcvs"
  In1/1 -> Product/1  "a"
  Bus Creator1/1 -> dxcvs1/1  "dxcvs"
  Demux1/3 -> Bus Creator1/3
  Demux1/2 -> Bus Creator1/2
  Demux1/1 -> Bus Creator1/1
  Demux1/10 -> Bus Creator1/10
  Demux1/9 -> Bus Creator1/9
  Demux1/4 -> Bus Creator1/4
  Bus to Vector/1 -> Product/2
  Product/1 -> Demux1/1
  Demux1/5 -> Bus Creator1/5
  Demux1/7 -> Bus Creator1/7
  Demux1/8 -> Bus Creator1/8
  Demux1/6 -> Bus Creator1/6

== system patient_model/cvs integrator/Subsystem3 ==
  In1 : Inport  OutDataTypeStr=Bus: CardioVascularStateDerivative
  Enable : EnablePort
  Out1 : Outport  OutDataTypeStr=Bus: CardioVascularStateDerivative
  wires:
  In1/1 -> Out1/1

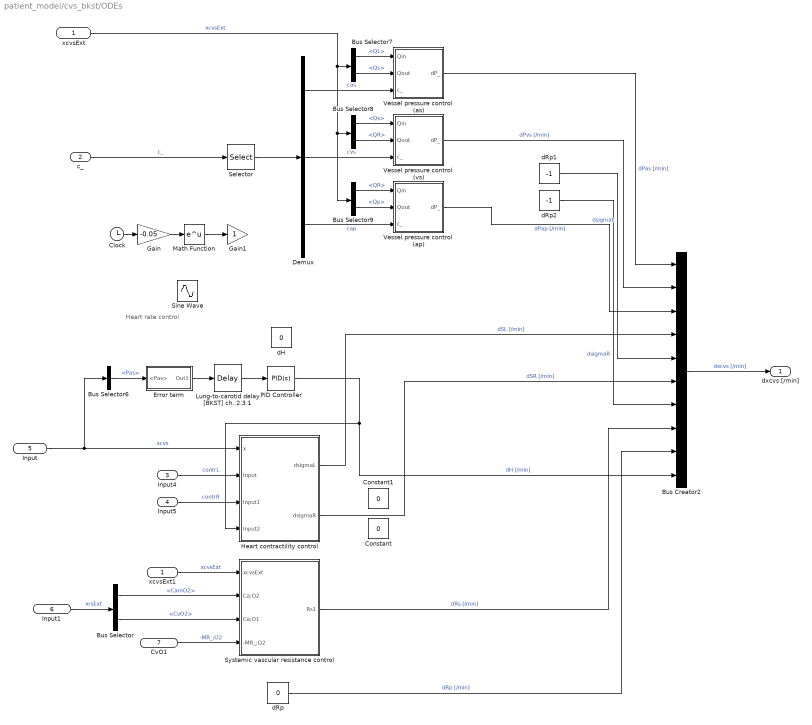
== system patient_model/cvs_bkst/ODEs ==
  note: Heart rate control
  xcvsExt : Inport  OutDataTypeStr=Bus: CardioVascularStateExtended
  c_ : Inport  Port=2  Unit=L/mmHg
  Input4 : Inport  Port=3  OutDataTypeStr=double  PortDimensions=3
  Input5 : Inport  Port=4  OutDataTypeStr=double  PortDimensions=3
  Input : Inport  Port=5  OutDataTypeStr=Bus: CardioVascularState
  Input1 : Inport  Port=6  OutDataTypeStr=Bus: RespiratoryStateExtended
  CvO1 : Inport  Port=7  Unit=L/min
  Bus Creator2 : BusCreator  Inputs=10  OutDataTypeStr=Bus: CardioVascularStateDerivative
  Bus Selector : BusSelector  OutputSignals=CamO2,CvO2
  Bus Selector6 : BusSelector  OutputSignals=Pas
  Bus Selector7 : BusSelector  OutputSignals=QL,Qs
  Bus Selector8 : BusSelector  OutputSignals=Qs,QR
  Bus Selector9 : BusSelector  OutputSignals=QR,Qp
  Clock : Clock
  Constant : Constant  Value=0
  Constant1 : Constant  Value=0
  Demux : Demux  Outputs=3
  Error term : Subsystem
  Gain : Gain  Gain=-0.05
  Gain1 : Gain
  Heart contractility control : Subsystem
  Lung-to-carotid delay [BKST] ch. 2.3.1 : TransportDelay  DelayTime=6
  Math Function : Math  SignedPower=off  SaturateOnIntegerOverflow=on
  PID Controller : simulink/Continuous/PID Controller  Controller=PID  Form=Parallel  TimeDomain=Continuous-time  SampleTime=-1  IntegratorMethod=Forward Euler  FilterMethod=Forward Euler  ControllerParametersSource=internal  P=1  I=0  D=-1  UseFilter=on  N=100  TunerSelectOption=Transfer Function Based (PID Tuner App)  InitialConditionSource=internal  InitialConditionForIntegrator=0  InitialConditionForFilter=0  DifferentiatorICPrevScaledInput=0  ExternalReset=none  TrackingMode=off  Kt=1  LimitOutput=off  UpperSaturationLimit=inf  LowerSaturationLimit=-inf  LinearizeAsGain=on  AntiWindupMode=none  Kb=1  POutMin=[]  POutMax=[]  IOutMin=[]  IOutMax=[]  DOutMin=[]  DOutMax=[]  NOutMin=[]  NOutMax=[]  SumOutMin=[]  SumOutMax=[]  SaturationOutMin=[]  SaturationOutMax=[]  PParamMin=[]  PParamMax=[]  IParamMin=[]  IParamMax=[]  DParamMin=[]  DParamMax=[]  NParamMin=[]  NParamMax=[]  KbParamMin=[]  KbParamMax=[]  KtParamMin=[]  KtParamMax=[]  KbOutMin=[]  KbOutMax=[]  KtOutMin=[]  KtOutMax=[]  IntegratorOutMin=[]  IntegratorOutMax=[]  FilterOutMin=[]  FilterOutMax=[]  SumI1OutMin=[]  SumI1OutMax=[]  SumI2OutMin=[]  SumI2OutMax=[]  SumI3OutMin=[]  SumI3OutMax=[]  SumI4OutMin=[]  SumI4OutMax=[]  SumDOutMin=[]  SumDOutMax=[]  DifferentiatorOutMin=[]  DifferentiatorOutMax=[]  FilterDiffOutCoefMin=[]  FilterDiffOutCoefMax=[]  ReciprocalOutMin=[]  ReciprocalOutMax=[]  SumDenOutMin=[]  SumDenOutMax=[]  SumNumOutMin=[]  SumNumOutMax=[]  DivideOutMin=[]  DivideOutMax=[]  IntegratorContinuousStateAttributes=''  IntegratorStateMustResolveToSignalObject=off  IntegratorRTWStateStorageClass=Auto  FilterContinuousStateAttributes=''  FilterStateMustResolveToSignalObject=off  FilterRTWStateStorageClass=Auto  ParallelPVariant=InternalParameters  IdealPVariant=Disabled  IVariant=InternalParameters  DVariant=InternalParameters  IntegratorVariant=Continuous  SatVariant=Disabled  AWVariant=Passthrough  PCopyVariant=Disabled  TRVariant=Disabled  FdbkBlocksVariant=Forward  IdealPFdbkVariant=Disabled  SatFdbkVariant=Disabled  DerivativeFilterVariant=ContFilter  NVariant=InternalParameters  NCopyVariant=Disabled  FilterICVariant=InternalICsFilter  IntegratorICVariant=InternalICs  ExternalResetVariant=Disabled  TRSumVariant=Passthrough  SumFdbkVariant=Disabled  SumVariant=Sum_PID
  Selector : Selector  InputPortWidth=4  IndexOptions=Index vector (dialog)  Indices=[1 2 3]  OutputSizes=1
  Sine Wave : Sin  Amplitude=0.4  Frequency=0.05  SampleTime=0
  Systemic vascular resistance control : Subsystem
  Vessel pressure control (ap) : Subsystem
  Vessel pressure control (as) : Subsystem
  Vessel pressure control (vs) : Subsystem
  dH : Constant  Value=0
  dRp : Constant  Value=0
  dRp1 : Constant  Value=-1
  dRp2 : Constant  Value=-1
  xcvsExt1 : InportShadow  OutDataTypeStr=Bus: CardioVascularStateExtended
  dxcvs [/min] : Outport  OutDataTypeStr=Bus: CardioVascularStateDerivative
  wires:
  Error term/1(Out1) -> Lung-to-carotid delay [BKST] ch. 2.3.1/1
  Bus Selector/2 -> Systemic vascular resistance control/3(Ca;O1)  "<CvO2>"
  Bus Selector8/2 -> Vessel pressure control (vs)/2(Qout)  "<QR>"
  Input1/1 -> Bus Selector/1  "xrsExt"
  Bus Selector/1 -> Systemic vascular resistance control/2(Ca;O2)  "<CamO2>"
  Bus Selector7/1 -> Vessel pressure control (as)/1(Qin)  "<QL>"
  Bus Selector7/2 -> Vessel pressure control (as)/2(Qout)  "<Qs>"
  Bus Creator2/1 -> dxcvs [/min]/1  "dxcvs [/min]"
  Selector/1 -> Demux/1
  Demux/3 -> Vessel pressure control (ap)/3(c_)  "cap"
  Clock/1 -> Gain/1
  Bus Selector9/2 -> Vessel pressure control (ap)/2(Qout)  "<Qp>"
  Input5/1 -> Heart contractility control/3(Input1)  "contrR"
  dRp1/1 -> Bus Creator2/5  "dsigmaL"
  Heart contractility control/2(dsigmaR) -> Bus Creator2/6  "dSR [/min]"
  PID Controller/1 -> Bus Creator2/10, Heart contractility control/4(Input2)  "dH [/min]"
  Input4/1 -> Heart contractility control/2(Input)  "contrL"
  Input/1 -> Bus Selector6/1, Heart contractility control/1(x)  "xcvs"
  xcvsExt1/1 -> Systemic vascular resistance control/1(xcvsExt)  "xcvsExt"
  Math Function/1 -> Gain1/1
  dRp2/1 -> Bus Creator2/7  "dsigmaR"
  xcvsExt/1 -> Bus Selector7/1, Bus Selector8/1, Bus Selector9/1  "xcvsExt"
  dRp/1 -> Bus Creator2/9  "dRp [/min]"
  Systemic vascular resistance control/1(Rs1) -> Bus Creator2/8  "dRs [/min]"
  Demux/1 -> Vessel pressure control (as)/3(c_)  "cas"
  Vessel pressure control (as)/1(dP_) -> Bus Creator2/1  "dPas [/min]"
  Heart contractility control/1(dsigmaL) -> Bus Creator2/4  "dSL [/min]"
  c_/1 -> Selector/1  "c_"
  Bus Selector9/1 -> Vessel pressure control (ap)/1(Qin)  "<QR>"
  Demux/2 -> Vessel pressure control (vs)/3(c_)  "cvs"
  CvO1/1 -> Systemic vascular resistance control/4(-MR_;O2)  "-MR_;O2"
  Gain/1 -> Math Function/1
  Lung-to-carotid delay [BKST] ch. 2.3.1/1 -> PID Controller/1
  Vessel pressure control (vs)/1(dP_) -> Bus Creator2/2  "dPvs [/min]"
  Bus Selector6/1 -> Error term/1(<Pas>)  "<Pas>"
  Bus Selector8/1 -> Vessel pressure control (vs)/1(Qin)  "<Qs>"
  Vessel pressure control (ap)/1(dP_) -> Bus Creator2/3  "dPap [/min]"

== system patient_model/rs integrator/Subsystem ==
  In1 : Inport
  dxcvs : Inport  Port=2
  Bus Creator1 : BusCreator  Inputs=6  OutDataTypeStr=Bus: RespiratoryStateDerivative
      settings: InheritFromInputs=off
  Bus to Vector : BusToVector
  Demux1 : Demux  Outputs=6
  Product : Product
  dxcvs1 : Outport
  wires:
  Demux1/6 -> Bus Creator1/6
  Demux1/5 -> Bus Creator1/5
  Demux1/4 -> Bus Creator1/4
  Demux1/3 -> Bus Creator1/3
  Demux1/2 -> Bus Creator1/2
  Demux1/1 -> Bus Creator1/1
  dxcvs/1 -> Bus to Vector/1  "dxrs"
  In1/1 -> Product/1  "a"
  Bus Creator1/1 -> dxcvs1/1  "dxrs"
  Bus to Vector/1 -> Product/2
  Product/1 -> Demux1/1

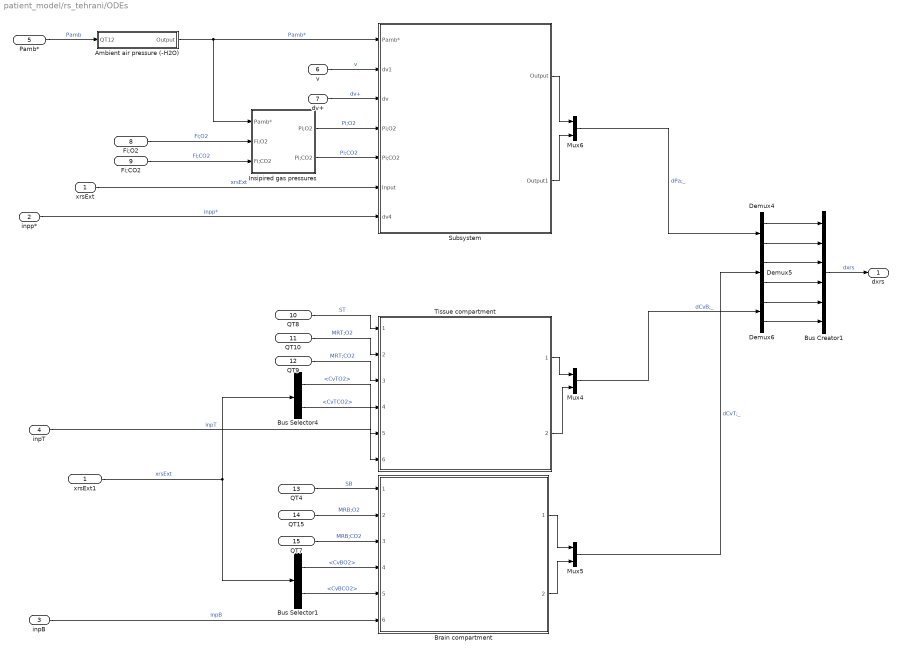
== system patient_model/rs_tehrani/ODEs ==
  xrsExt : Inport  OutDataTypeStr=Bus: RespiratoryStateExtended
  inpp* : Inport  Port=2  OutDataTypeStr=Bus: BloodGasFlow
  inpB : Inport  Port=3  OutDataTypeStr=Bus: BloodGasFlow
  inpT : Inport  Port=4  OutDataTypeStr=Bus: BloodGasFlow
  Pamb* : Inport  Port=5  Unit=mmHg
  v : Inport  Port=6  Unit=L
  dv+ : Inport  Port=7  Unit=L/s
  Fi;O2 : Inport  Port=8  Unit=1
  Fi;CO2 : Inport  Port=9  Unit=1
  QT8 : Inport  Port=10  Unit=L
  QT10 : Inport  Port=11  Unit=L/s
  QT9 : Inport  Port=12  Unit=L/s
  QT4 : Inport  Port=13  Unit=L
  QT15 : Inport  Port=14  Unit=L/s
  QT7 : Inport  Port=15  Unit=L/s
  Ambient air pressure (-H2O) : Subsystem  TreatAsAtomicUnit=on
  Brain compartment : Subsystem  ReferencedSubsystem=tehrani_tissue_compartment_v2
  Bus Creator1 : BusCreator  Inputs=6  OutDataTypeStr=Bus: RespiratoryStateDerivative
      settings: InheritFromInputs=off
  Bus Selector1 : BusSelector  OutputSignals=CvBO2,CvBCO2
  Bus Selector4 : BusSelector  OutputSignals=CvTO2,CvTCO2
  Demux4 : Demux  Outputs=2
  Demux5 : Demux  Outputs=2
  Demux6 : Demux  Outputs=2
  Insipired gas pressures : Subsystem  TreatAsAtomicUnit=on
  Mux4 : Mux  Inputs=2
  Mux5 : Mux  Inputs=2
  Mux6 : Mux  Inputs=2
  Subsystem : Subsystem
  Tissue compartment : Subsystem  ReferencedSubsystem=tehrani_tissue_compartment_v2
  xrsExt1 : InportShadow  OutDataTypeStr=Bus: RespiratoryStateExtended
  dxrs : Outport  OutDataTypeStr=Bus: RespiratoryStateDerivative
  wires:
  Subsystem/2(Output1) -> Mux6/2
  Subsystem/1(Output) -> Mux6/1
  inpp*/1 -> Subsystem/7(dv4)  "inpp*"
  xrsExt/1 -> Subsystem/6(Input)  "xrsExt"
  Insipired gas pressures/2(Pi;CO2) -> Subsystem/5(Pi;CO2)  "Pi;CO2"
  Insipired gas pressures/1(Pi;O2) -> Subsystem/4(Pi;O2)  "Pi;O2"
  dv+/1 -> Subsystem/3(dv)  "dv+"
  v/1 -> Subsystem/2(dv1)  "v"
  Bus Creator1/1 -> dxrs/1  "dxrs"
  inpB/1 -> Brain compartment/6  "inpB"
  Bus Selector4/2 -> Tissue compartment/5  "<CvTCO2>"
  Mux4/1 -> Demux6/1  "dCvB;_"
  Bus Selector4/1 -> Tissue compartment/4  "<CvTO2>"
  QT8/1 -> Tissue compartment/1  "ST"
  Brain compartment/2 -> Mux5/2
  Mux6/1 -> Demux4/1  "dPa;_"
  inpT/1 -> Tissue compartment/6  "inpT"
  Brain compartment/1 -> Mux5/1
  Mux5/1 -> Demux5/1  "dCvT;_"
  Demux6/2 -> Bus Creator1/6
  QT10/1 -> Tissue compartment/2  "MRT;O2"
  Demux5/2 -> Bus Creator1/4
  Demux6/1 -> Bus Creator1/5
  Tissue compartment/1 -> Mux4/1
  Demux5/1 -> Bus Creator1/3
  Tissue compartment/2 -> Mux4/2
  QT9/1 -> Tissue compartment/3  "MRT;CO2"
  Pamb*/1 -> Ambient air pressure (-H2O)/1(QT12)  "Pamb"
  Demux4/1 -> Bus Creator1/1
  QT7/1 -> Brain compartment/3  "MRB;CO2"
  Bus Selector1/1 -> Brain compartment/4  "<CvBO2>"
  Fi;CO2/1 -> Insipired gas pressures/3(Fi;CO2)  "Fi;CO2"
  QT4/1 -> Brain compartment/1  "SB"
  QT15/1 -> Brain compartment/2  "MRB;O2"
  Demux4/2 -> Bus Creator1/2
  Ambient air pressure (-H2O)/1(Output) -> Insipired gas pressures/1(Pamb*), Subsystem/1(Pamb*)  "Pamb*"
  Bus Selector1/2 -> Brain compartment/5  "<CvBCO2>"
  Fi;O2/1 -> Insipired gas pressures/2(Fi;O2)  "Fi;O2"
  xrsExt1/1 -> Bus Selector4/1, Bus Selector1/1  "xrsExt"

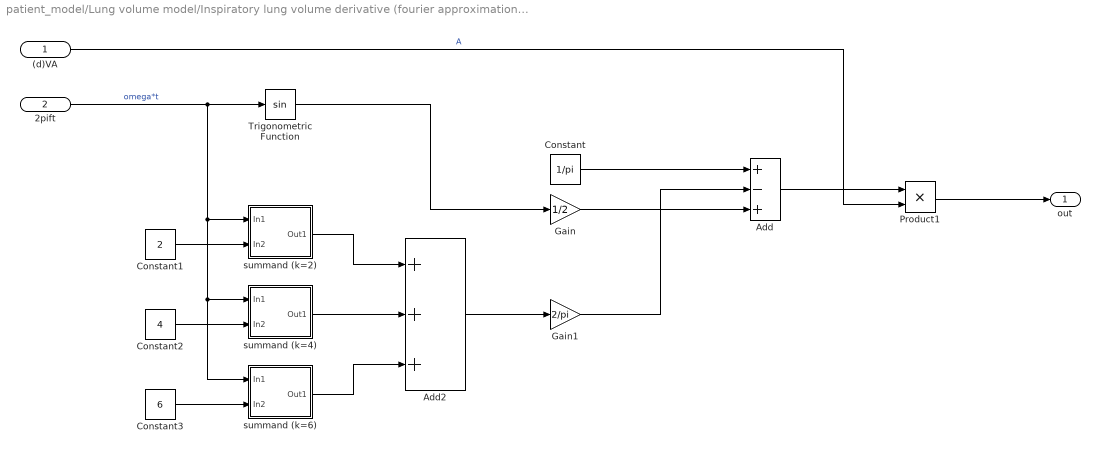
== system patient_model/Lung volume model/Inspiratory lung volume derivative (fourier approximation)/Half-wave rectifier ==
  (d)VA : Inport
  2pift : Inport  Port=2
  Add : Sum  Inputs=+-+
  Add2 : Sum  Inputs=+++
  Constant : Constant  Value=1/pi
  Constant1 : Constant  Value=2
  Constant2 : Constant  Value=4
  Constant3 : Constant  Value=6
  Gain : Gain  Gain=1/2
  Gain1 : Gain  Gain=2/pi
  Product1 : Product
  Trigonometric Function : Trigonometry
  summand (k=2) : Subsystem
  summand (k=4) : Subsystem
  summand (k=6) : Subsystem
  out : Outport
  wires:
  Constant2/1 -> summand (k=4)/2(In2)
  Constant3/1 -> summand (k=6)/2(In2)
  summand (k=6)/1(Out1) -> Add2/3
  summand (k=4)/1(Out1) -> Add2/2
  summand (k=2)/1(Out1) -> Add2/1
  Constant1/1 -> summand (k=2)/2(In2)
  Add2/1 -> Gain1/1
  Gain1/1 -> Add/2
  Product1/1 -> out/1
  Add/1 -> Product1/1
  Constant/1 -> Add/1
  2pift/1 -> Trigonometric Function/1, summand (k=2)/1(In1), summand (k=4)/1(In1), summand (k=6)/1(In1)  "omega*t"
  (d)VA/1 -> Product1/2  "A"
  Gain/1 -> Add/3
  Trigonometric Function/1 -> Gain/1

== system patient_model/Predicted Body Weight1/IfThenElse/Subsystem1 ==
  in : Inport
  Enable : EnablePort
  out : Outport
  wires:
  in/1 -> out/1

== system patient_model/Predicted Body Weight1/IfThenElse/Subsystem2 ==
  in : Inport
  Enable : EnablePort
  out : Outport
  wires:
  in/1 -> out/1

== system patient_model/cvs_bkst/ODEs/Error term ==
  <Pas> : Inport  Unit=mmHg
  Pas^ : Constant  Value=100
  Subtract : Sum  Inputs=-+
  Out1 : Outport
  wires:
  Subtract/1 -> Out1/1  "s"
  Pas^/1 -> Subtract/2
  <Pas>/1 -> Subtract/1  "Pas"

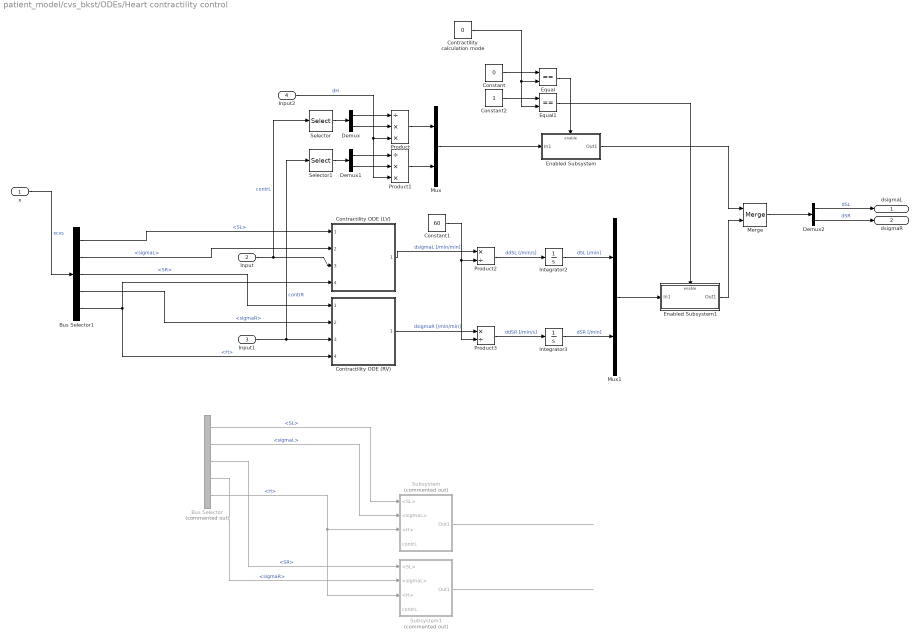
== system patient_model/cvs_bkst/ODEs/Heart contractility control ==
  x : Inport  OutDataTypeStr=Bus: CardioVascularState
  Input : Inport  Port=2  OutDataTypeStr=double  PortDimensions=3
  Input1 : Inport  Port=3  OutDataTypeStr=double  PortDimensions=3
  Input2 : Inport  Port=4  Unit=1/min^2
  Bus Selector : BusSelector  Commented=on  OutputSignals=SL,sigmaL,SR,sigmaR,H
  Bus Selector1 : BusSelector  OutputSignals=SL,sigmaL,SR,sigmaR,H
  Constant : Constant  Value=0
  Constant1 : Constant  Value=60
  Constant2 : Constant
  Contractility ODE (LV) : Subsystem  ReferencedSubsystem=cvrs_contractility_control
  Contractility ODE (RV) : Subsystem  ReferencedSubsystem=cvrs_contractility_control
  Contractility calculation mode : Constant  Value=0
  Demux : Demux  Outputs=2
  Demux1 : Demux  Outputs=2
  Demux2 : Demux  Outputs=2
  Enabled Subsystem : Subsystem  TreatAsAtomicUnit=on
  Enabled Subsystem1 : Subsystem  TreatAsAtomicUnit=on
  Equal : RelationalOperator  Operator===  OutDataTypeStr=boolean  RndMeth=Simplest
  Equal1 : RelationalOperator  Operator===  OutDataTypeStr=boolean  RndMeth=Simplest
  Integrator2 : Integrator
  Integrator3 : Integrator
  Merge : Merge
  Mux : Mux  Inputs=2
  Mux1 : Mux  Inputs=2
  Product : Product  Inputs=/**
  Product1 : Product  Inputs=/**
  Product2 : Product  Inputs=*/
  Product3 : Product  Inputs=*/
  Selector : Selector  InputPortWidth=3  IndexOptions=Index vector (dialog)  Indices=[1 2]  OutputSizes=1
  Selector1 : Selector  InputPortWidth=3  IndexOptions=Index vector (dialog)  Indices=[1 2]  OutputSizes=1
  Subsystem : Subsystem  Commented=on
  Subsystem1 : Subsystem  Commented=on
  dsigmaL : Outport  Unit=mmHg/min
  dsigmaR : Outport  Port=2  Unit=mmHg/min
  wires:
  Input2/1 -> Product/3, Product1/3  "dH"
  Contractility calculation mode/1 -> Equal/2, Equal1/2
  Constant2/1 -> Equal1/1
  Constant/1 -> Equal/1
  Merge/1 -> Demux2/1
  Demux2/2 -> dsigmaR/1  "dSR"
  Demux2/1 -> dsigmaL/1  "dSL"
  Enabled Subsystem1/1(Out1) -> Merge/2
  Enabled Subsystem/1(Out1) -> Merge/1
  Equal1/1 -> Enabled Subsystem1/Enable
  Equal/1 -> Enabled Subsystem/Enable
  Mux1/1 -> Enabled Subsystem1/1(In1)
  Mux/1 -> Enabled Subsystem/1(In1)
  Product1/1 -> Mux/2
  Product/1 -> Mux/1
  Selector1/1 -> Demux1/1
  Demux1/1 -> Product1/1
  Demux1/2 -> Product1/2
  Demux/2 -> Product/2
  Demux/1 -> Product/1
  Selector/1 -> Demux/1
  Bus Selector/4 -> Subsystem1/2(<sigmaL>)  "<sigmaR>"
  Bus Selector/3 -> Subsystem1/1(<SL>)  "<SR>"
  Subsystem1/1(Out1) -> ?
  Subsystem/1(Out1) -> ?
  ? -> Subsystem/4(contrL)  "contrL"
  Bus Selector/5 -> Subsystem/3(<H>), Subsystem1/3(<H>)  "<H>"
  Bus Selector/2 -> Subsystem/2(<sigmaL>)  "<sigmaL>"
  Bus Selector/1 -> Subsystem/1(<SL>)  "<SL>"
  Bus Selector1/5 -> Contractility ODE (RV)/4, Contractility ODE (LV)/4  "<H>"
  Bus Selector1/2 -> Contractility ODE (LV)/2  "<sigmaL>"
  Bus Selector1/4 -> Contractility ODE (RV)/2  "<sigmaR>"
  x/1 -> Bus Selector1/1  "xcvs"
  Contractility ODE (RV)/1 -> Product3/1  "dsigmaR [/min/min]"
  Bus Selector1/1 -> Contractility ODE (LV)/1  "<SL>"
  Input/1 -> Selector/1, Contractility ODE (LV)/3  "contrL"
  Contractility ODE (LV)/1 -> Product2/1  "dsigmaL [/min/min]"
  Input1/1 -> Contractility ODE (RV)/3, Selector1/1  "contrR"
  Bus Selector1/3 -> Contractility ODE (RV)/1  "<SR>"
  Constant1/1 -> Product3/2, Product2/2
  Product2/1 -> Integrator2/1  "ddSL [/min/s]"
  Product3/1 -> Integrator3/1  "ddSR [/min/s]"
  Integrator2/1 -> Mux1/1  "dSL [/min]"
  Integrator3/1 -> Mux1/2  "dSR [/min]"
  ? -> Subsystem1/4(contrL)  "contrR"
  ? -> Bus Selector/1  "xcvs"

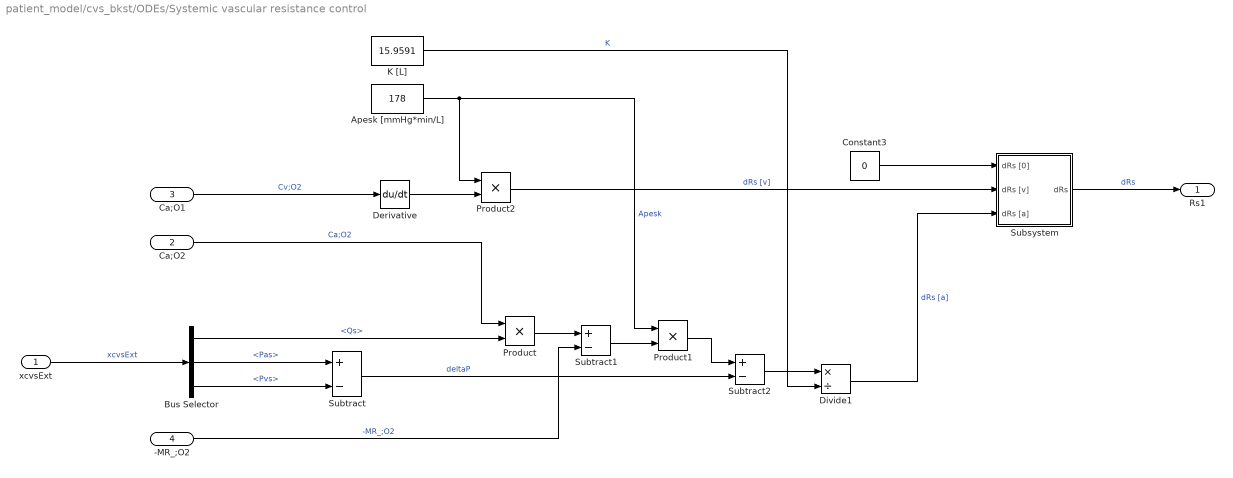
== system patient_model/cvs_bkst/ODEs/Systemic vascular resistance control ==
  xcvsExt : Inport  OutDataTypeStr=Bus: CardioVascularStateExtended
  Ca;O2 : Inport  Port=2  Unit=1
  Ca;O1 : Inport  Port=3  Unit=1
  -MR_;O2 : Inport  Port=4  Unit=L/min
  Apesk [mmHg*min/L] : Constant  Value=178
  Bus Selector : BusSelector  OutputSignals=Qs,Pas,Pvs
  Constant3 : Constant  Value=0
  Derivative : Derivative
  Divide1 : Product  Inputs=*/
  K [L] : Constant  Value=15.9591
  Product : Product
  Product1 : Product
  Product2 : Product
  Subsystem : Subsystem
  Subtract : Sum  Inputs=+-
  Subtract1 : Sum  Inputs=+-
  Subtract2 : Sum  Inputs=+-
  Rs1 : Outport  Unit=mmHg/L
  wires:
  Subsystem/1(dRs) -> Rs1/1  "dRs"
  Divide1/1 -> Subsystem/3(dRs [a])  "dRs [a]"
  Product2/1 -> Subsystem/2(dRs [v])  "dRs [v]"
  Constant3/1 -> Subsystem/1(dRs [0])
  Derivative/1 -> Product2/2
  Ca;O1/1 -> Derivative/1  "Cv;O2"
  Bus Selector/3 -> Subtract/2  "<Pvs>"
  xcvsExt/1 -> Bus Selector/1  "xcvsExt"
  K [L]/1 -> Divide1/2  "K"
  Apesk [mmHg*min/L]/1 -> Product1/1, Product2/1  "Apesk"
  Bus Selector/1 -> Product/2  "<Qs>"
  Bus Selector/2 -> Subtract/1  "<Pas>"
  Ca;O2/1 -> Product/1  "Ca;O2"
  Subtract/1 -> Subtract2/2  "deltaP"
  Subtract1/1 -> Product1/2
  Subtract2/1 -> Divide1/1
  Product/1 -> Subtract1/1
  Product1/1 -> Subtract2/1
  -MR_;O2/1 -> Subtract1/2  "-MR_;O2"
